simulink library "CampusModeling"  (Simulink 7.8)
settings: Solver=ode45  StartTime=0.0  StopTime=10.0  RelTol=1e-3
settings Model: Creator=sfrank1  LastModifiedBy=wbernal

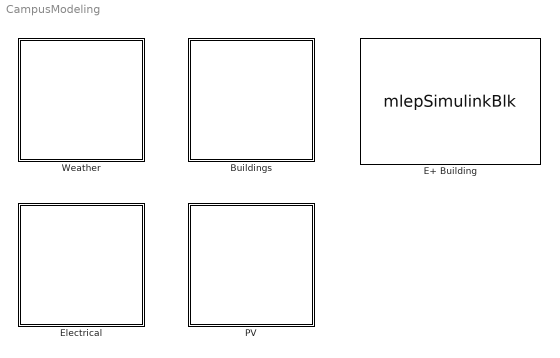
== system CampusModeling ==
  Buildings : Subsystem  Tag=Weather  Description=Contains blocks for acquiring and manipulating weather data.
      mask Display: disp('Buildings')
  E+ Building : M-S-Function  FunctionName=mlepSimulinkBlk  Parameters=progname, modelfile, weatherfile, workdir, timeout, port, host, bcvtbdir, deltaT, noutputd  mask(EnergyPlus Cosimulation){progname='C:\\EnergyPlusV8-0-0-mlep\\RunEPlus.bat', modelfile='U:\\Simulink-mlep\\Hospital\\RefBldgHospitalNew2004_Chicago', weatherfile='USA_IL_Chicago-OHare.Intl.AP.725300_TMY3', workdir='U:\\Simulink-mlep\\Hospital', timeout=80000, port=0, host='', bcvtbdir='', deltaT=900, noutputd=2}
      mask prompts: progname "E+ Executable Path"; modelfile "IDF File (without extension)"; weatherfile "Weather Profile"; workdir "Working Directory"; timeout "Timeout (in milliseconds)"; port "Socket Port (0 = any available)"; host "Socket Host ('' = local host)"; bcvtbdir "BCVTB Directory"; deltaT "Time Step (in seconds)"; noutputd "Number of Real Outputs"
      mask help: This block implements cosimulation with EnergyPlus by allowing Simulink to exchange input and output data with it. Currently, EnergyPlus only supports real data.
      mask Help:
      | This block implements cosimulation with EnergyPlus by allowing Simulink to
      | exchange input and output data with it.
      | 
      | When a simulation starts, EnergyPlus is also started. It will then run in
      | parallel with Simulink. They exchange input and output data via socket
      | communication. When the simulation terminates, EnergyPlus will exit.
      | 
      | Refer to the manuals of MLE+ and/or BCVTB/EnergyPlus for details.
      | 
      | INPUTS:
      | - real: real vector input to EnergyPlus.
      | 
      | OUTPUTS:
      | - flag: status of EnergyPlus (0 if OK, if flag is non-zero, the simulation should stop).
      | - time: current simulation time of EnergyPlus, in seconds.
      | - real: real vector output from EnergyPlus.
      mask Display:
      | disp('E+\nCosimulation');
      | port_label('output', 1, 'flag');
      | port_label('output', 2, 'time');
      | port_label('output', 3, 'real');
      | % port_label('output', 4, 'int');
      | % port_label('output', 5, 'bool');
      | port_label('input', 1, 'real');
      | % port_label('input', 2, 'int');
      | % port_label('input', 3, 'bool');
      | image(imread('building.png'))
  Electrical : Subsystem  Tag=Weather  Description=Contains blocks for acquiring and manipulating weather data.
      mask Display: disp('Electrical')
  PV : Subsystem  Tag=Weather  Description=Contains blocks for acquiring and manipulating weather data.
      mask Display: disp('PV')
  Weather : Subsystem  Tag=Weather  Description=Contains blocks for acquiring and manipulating weather data.
      mask Display: disp('Weather')

== system CampusModeling/Buildings ==

== system CampusModeling/Electrical ==

== system CampusModeling/PV ==

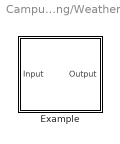
== system CampusModeling/Weather ==
  Example : Subsystem  mask{gain=2}
      mask prompts: gain "Enter a gain"
      mask help: Example custom library block. Applies a user-specified gain to the input signal.
      mask Help: Example custom library block. Applies a user-specified gain to the input signal.
      mask Display: plot([0.8 -1 -1 0 -1 -1 0.8],[1 1 0 0 0 -1 -1],4,4,-4,-4)

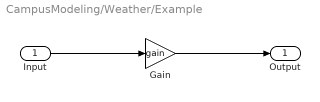
== system CampusModeling/Weather/Example ==
  Input : Inport
  Gain : Gain  Gain=gain
  Output : Outport
  wires:
  Input/1 -> Gain/1
  Gain/1 -> Output/1
